simulink model "SimuleringRegAfl1"  (R2021b)
settings: Solver=VariableStepAuto  StartTime=0.0  StopTime=10.0  RelTol=1e-3
values from neighbouring files (symbols this model uses):
  b = 0.1    [handinTemplate.m]
  g = 9.82    [handinTemplate.m]
  Kp = 1    [Portfolio_1_Modeling_and_Control_of_Robot_Arm.m]    (also in dotxPidController.m = 0.5 * Model.Tp / (Model.Tdt*Model.K); handinTemplate.m = 0.97; port1.m = 85)
  l = 0.5    [handinTemplate.m]
  m = 1    [handinTemplate.m]
  N = 10    [Portfolio_1_Modeling_and_Control_of_Robot_Arm.m]    (also in handinTemplate.m; port1.m = 20)
  Td = 1/5    (= 0.2)    [Portfolio_1_Modeling_and_Control_of_Robot_Arm.m]    (also in dotxPidController.m = 0.5*Model.Tdt; handinTemplate.m; port1.m = 0.142857142857)
  Ti = 1    [Portfolio_1_Modeling_and_Control_of_Robot_Arm.m]    (also in dotxPidController.m = min( 8*Model.Tdt, Model.Tp); handinTemplate.m; port1.m)
undefined symbols (not defined in the file or in its folder): I
libraries: slpidlib x1
settings Model: Creator=nvigg  LastModifiedBy=Thomas Therkelsen
settings SolverCC: AlgebraicLoopSolver=TrustRegion
settings DebuggingCC: SFMachineParentedDataDiag=warning

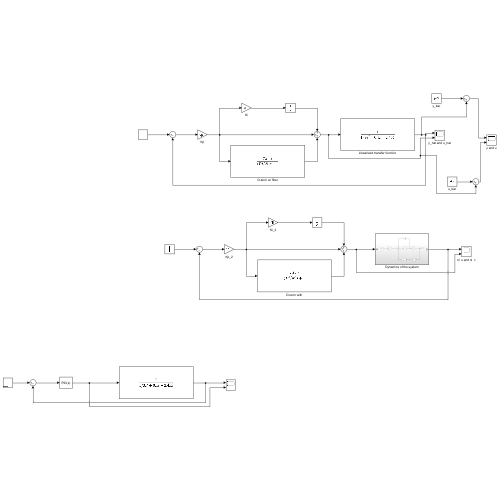
[thumbnail: Simulink's stored preview of the top-level diagram]
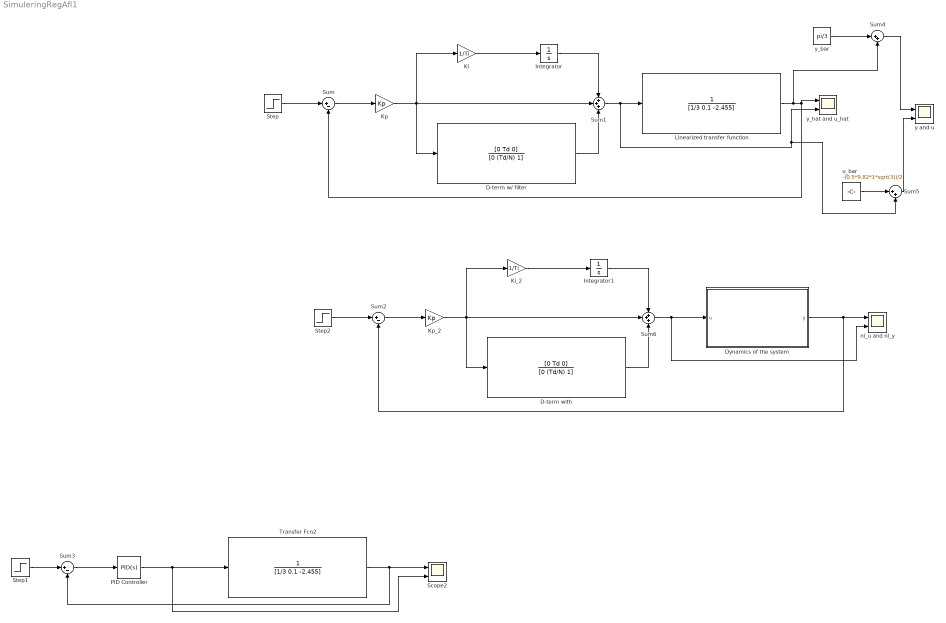
== system SimuleringRegAfl1 ==
  D-term w/ filter : TransferFcn  Numerator=[0 Td 0]  Denominator=[0 (Td/N) 1]
  D-term with : TransferFcn  Numerator=[0 Td 0]  Denominator=[0 (Td/N) 1]
  Dynamics of the system : Subsystem
  Integrator : Integrator
  Integrator1 : Integrator
  Ki : Gain  Gain=1/Ti
  Ki_2 : Gain  Gain=1/Ti
  Kp : Gain  Gain=Kp
  Kp_2 : Gain  Gain=Kp
  Linearized transfer function : TransferFcn  Denominator=[1/3 0.1 -2.455]
  PID Controller : slpidlib/PID Controller  Controller=PID  Form=Ideal  TimeDomain=Continuous-time  UseExternalTs=off  SampleTime=-1  IntegratorMethod=Forward Euler  FilterMethod=Forward Euler  ControllerParametersSource=internal  P=Kp  I=Ti  D=Td  UseFilter=on  N=N  TunerSelectOption=Transfer Function Based (PID Tuner App)  InitialConditionSource=internal  InitialConditionForIntegrator=0  InitialConditionForFilter=0  DifferentiatorICPrevScaledInput=0  ExternalReset=none  TrackingMode=off  Kt=1  LimitOutput=off  SatLimitsSource=internal  UpperSaturationLimit=inf  LowerSaturationLimit=-inf  LinearizeAsGain=on  AntiWindupMode=none  Kb=1  POutMin=[]  POutMax=[]  IOutMin=[]  IOutMax=[]  DOutMin=[]  DOutMax=[]  NOutMin=[]  NOutMax=[]  SumOutMin=[]  SumOutMax=[]  SaturationOutMin=[]  SaturationOutMax=[]  PParamMin=[]  PParamMax=[]  IParamMin=[]  IParamMax=[]  DParamMin=[]  DParamMax=[]  NParamMin=[]  NParamMax=[]  KbParamMin=[]  KbParamMax=[]  KtParamMin=[]  KtParamMax=[]  KbOutMin=[]  KbOutMax=[]  KtOutMin=[]  KtOutMax=[]  IntegratorOutMin=[]  IntegratorOutMax=[]  FilterOutMin=[]  FilterOutMax=[]  SumI1OutMin=[]  SumI1OutMax=[]  SumI2OutMin=[]  SumI2OutMax=[]  SumI3OutMin=[]  SumI3OutMax=[]  SumI4OutMin=[]  SumI4OutMax=[]  SumDOutMin=[]  SumDOutMax=[]  DifferentiatorOutMin=[]  DifferentiatorOutMax=[]  FilterDiffOutCoefMin=[]  FilterDiffOutCoefMax=[]  ReciprocalOutMin=[]  ReciprocalOutMax=[]  SumDenOutMin=[]  SumDenOutMax=[]  SumNumOutMin=[]  SumNumOutMax=[]  DivideOutMin=[]  DivideOutMax=[]  UdiffTsProdOutMin=[]  UdiffTsProdOutMax=[]  NTsProdOutMin=[]  NTsProdOutMax=[]  UintegralTsProdOutMin=[]  UintegralTsProdOutMax=[]  UngainTsProdOutMin=[]  UngainTsProdOutMax=[]  IntegratorContinuousStateAttributes=''  IntegratorStateMustResolveToSignalObject=off  IntegratorRTWStateStorageClass=Auto  FilterContinuousStateAttributes=''  FilterStateMustResolveToSignalObject=off  FilterRTWStateStorageClass=Auto  ParallelPVariant=Passthrough  IdealPVariant=InternalParameters  IVariant=InternalParameters  DVariant=InternalParameters  IntegratorVariant=Continuous  SatVariant=Disabled  AWVariant=Passthrough  PCopyVariant=Disabled  TRVariant=Disabled  FdbkBlocksVariant=Forward  IdealPFdbkVariant=Disabled  SatFdbkVariant=Disabled  DerivativeFilterVariant=ContFilter  NVariant=InternalParameters  NCopyVariant=Disabled  FilterICVariant=InternalICsFilter  IntegratorICVariant=InternalICs  ExternalResetVariant=Disabled  TRSumVariant=Passthrough  SumFdbkVariant=Disabled  SumVariant=Sum_PID  TsampFilterVariant=InternalTs  TsampNgainVariant=Passthrough  TsampIntegralVariant=Passthrough  ExternalSaturationOutDataTypeStr=Inherit: Same as second input
  Scope2 : Scope  NumInputPorts=2
  Step : Step  After=pi/3  SampleTime=0
  Step1 : Step  SampleTime=0
  Step2 : Step  After=pi/3  SampleTime=0
  Sum : Sum  Inputs=|+-
  Sum1 : Sum  Inputs=+++
  Sum2 : Sum  Inputs=|+-
  Sum3 : Sum  Inputs=|+-
  Sum4 : Sum  Inputs=|++
  Sum5 : Sum  Inputs=|++
  Sum6 : Sum  Inputs=+++
  Transfer Fcn2 : TransferFcn  Denominator=[1/3 0.1 -2.455]
  nl_u and nl_y : Scope  NumInputPorts=2
  u_bar : Constant  Value=-(0.5*9.82*1*sqrt(3))/2
  y and u : Scope  NumInputPorts=2
  y_bar : Constant  Value=pi/3
  y_hat and u_hat : Scope  NumInputPorts=2
  wires:
  Step/1 -> Sum/1
  Sum/1 -> Kp/1
  Kp/1 -> D-term w/ filter/1, Sum1/2, Ki/1
  Ki/1 -> Integrator/1
  Sum1/1 -> Sum5/2, y_hat and u_hat/2, Linearized transfer function/1
  Integrator/1 -> Sum1/1
  D-term w/ filter/1 -> Sum1/3
  Linearized transfer function/1 -> Sum4/2, Sum/2, y_hat and u_hat/1
  PID Controller/1 -> Scope2/2, Transfer Fcn2/1
  Sum3/1 -> PID Controller/1
  Step1/1 -> Sum3/1
  Transfer Fcn2/1 -> Sum3/2, Scope2/1
  y_bar/1 -> Sum4/1
  Sum4/1 -> y and u/1
  u_bar/1 -> Sum5/1
  Sum5/1 -> y and u/2
  Dynamics of the system/1(y) -> Sum2/2, nl_u and nl_y/1
  Ki_2/1 -> Integrator1/1
  Kp_2/1 -> D-term with/1, Sum6/2, Ki_2/1
  Sum2/1 -> Kp_2/1
  D-term with/1 -> Sum6/3
  Step2/1 -> Sum2/1
  Integrator1/1 -> Sum6/1
  Sum6/1 -> nl_u and nl_y/2, Dynamics of the system/1(u)

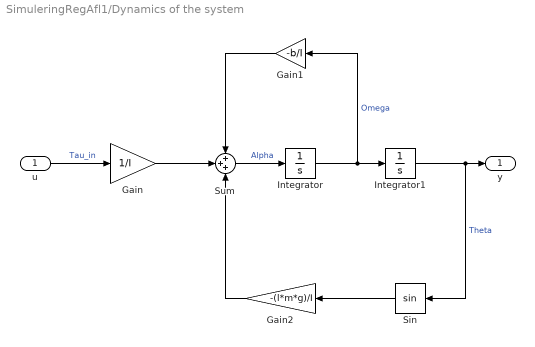
== system SimuleringRegAfl1/Dynamics of the system ==
  u : Inport
  Gain : Gain  Gain=1/I
  Gain1 : Gain  Gain=-b/I
  Gain2 : Gain  Gain=-(l*m*g)/I
  Integrator : Integrator
  Integrator1 : Integrator
  Sin : Trigonometry
  Sum : Sum  Inputs=+++
  y : Outport
  wires:
  u/1 -> Gain/1  "Tau_in"
  Gain/1 -> Sum/2
  Sum/1 -> Integrator/1  "Alpha"
  Integrator/1 -> Gain1/1, Integrator1/1  "Omega"
  Gain1/1 -> Sum/1
  Integrator1/1 -> Sin/1, y/1  "Theta"
  Gain2/1 -> Sum/3
  Sin/1 -> Gain2/1
